simulink model "NonControledLine12"  (R2015b)
settings: configuration reference "ControlConfig" (kept outside this file)
InitFcn:
  | ControlInit;
StopFcn:
  | PlotGridCode;
values from neighbouring files (symbols this model uses):
  c0 = c1/1000    (= 9.22e-13)    [ControlInit.m]
  c1 = 0.922e-9    (= 9.22e-10)    [ControlInit.m]
  Fnom = 50    [ControlInit.m]
  Grid_V = 400e3    (= 400000)    [ControlInit.m]
  L = Vl*Vl/(2*pi*fnom*S)    (= 0.0198943678865)    [XRCalculator.m]
  l0 = l1    (= 0.0013)    [ControlInit.m]
  l1 = 0.0013    [ControlInit.m]
  P_SP = 750e7    (= 7500000000)    [ControlInit.m]
  R = P/(Il*Il)    [XRCalculator.m]
  r0 = r1    (= 0.0731)    [ControlInit.m]
  r1 = 0.0731    [ControlInit.m]
  Ts = 0.02    [ControlInit.m]
  WtF_c0 = WtF_c1/1000    (= 9.22e-09)    [ControlInit.m]
  WtF_c1 = 0.922e-5    (= 9.22e-06)    [ControlInit.m]
  WtF_l0 = WtF_l1    (= 13000)    [ControlInit.m]
  WtF_l1 = 0.0013e7    (= 13000)    [ControlInit.m]
undefined symbols (not defined in the file or in its folder): DiscIntNeverNeededParam
libraries: powerlib x11, simulink x5, powerlib_meascontrol x2
settings Model: Creator=Emilio  LastModifiedBy=Emilio
settings ConfigSetRef: SourceLocation=Base Workspace

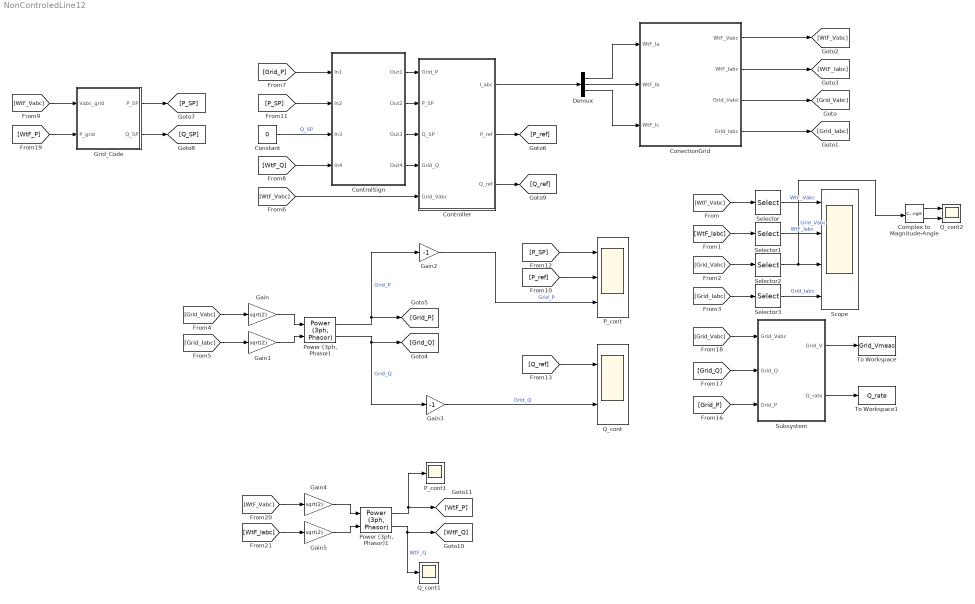
== system NonControledLine12 ==
  Complex to Magnitude-Angle : ComplexToMagnitudeAngle
  ConectionGrid : Subsystem
  Constant : Constant  Value=0
  ControlSign : Subsystem
  Controller : Subsystem
  Demux : Demux  Outputs=3
  Gain{,1,4..5} (4 alike) : Gain  Gain=sqrt(2)
  Gain2 : Gain  Gain=-1
  Gain3 : Gain  Gain=-1
  Grid_Code : Subsystem
  P_cont : Scope  NumInputPorts=3
  P_cont1 : Scope
  "Power (3ph, Phasor)" : powerlib_meascontrol/Measurements/Power (3ph, Phasor)
  "Power (3ph, Phasor)1" : powerlib_meascontrol/Measurements/Power (3ph, Phasor)
  Q_cont : Scope  NumInputPorts=2
  Q_cont1 : Scope
  Q_cont2 : Scope  NumInputPorts=2
  Scope : Scope  NumInputPorts=4
  Selector{,1..3} (4 alike) : Selector  InputPortWidth=3  IndexOptions=Index vector (dialog)  Indices=[1]  OutputSizes=1
  Subsystem : Subsystem
  To Workspace : ToWorkspace  VariableName=Grid_Vmeas  SampleTime=Ts
  To Workspace1 : ToWorkspace  VariableName=Q_rate  SampleTime=-1
  wires:
  ConectionGrid/1(WtF_Vabc) -> [WtF_Vabc]
  ConectionGrid/2(WtF_Iabc) -> [WtF_Iabc]
  ConectionGrid/3(Grid_Vabc) -> [Grid_Vabc]
  ConectionGrid/4(Grid_Iabc) -> [Grid_Iabc]
  [WtF_Vabc] -> Selector/1
  [WtF_Iabc] -> Selector1/1
  [Grid_Vabc] -> Selector2/1
  [Grid_Iabc] -> Selector3/1
  Selector/1 -> Scope/1  "WtF_Vabc"
  Selector1/1 -> Scope/2  "WtF_Iabc"
  Selector2/1 -> Complex to Magnitude-Angle/1, Scope/3  "Grid_Vabc"
  Selector3/1 -> Scope/4  "Grid_Iabc"
  [Grid_Vabc] -> Gain/1
  [Grid_Iabc] -> Gain1/1
  Gain/1 -> "Power (3ph, Phasor)"/1
  Gain1/1 -> "Power (3ph, Phasor)"/2
  "Power (3ph, Phasor)"/1 -> [Grid_P], Gain2/1  "Grid_P"
  "Power (3ph, Phasor)"/2 -> Gain3/1, [Grid_Q]  "Grid_Q"
  [WtF_Vabc] -> Controller/5(Grid_Vabc)
  Controller/1(I_abc) -> Demux/1
  Demux/1 -> ConectionGrid/1(WtF_Ia)
  Demux/2 -> ConectionGrid/2(WtF_Ib)
  Demux/3 -> ConectionGrid/3(WtF_Ic)
  [WtF_Vabc] -> Grid_Code/1(Vabc_grid)
  Gain2/1 -> P_cont/3  "Grid_P"
  Gain3/1 -> Q_cont/2  "Grid_Q"
  Controller/2(P_ref) -> [P_ref]
  [P_ref] -> P_cont/2
  Grid_Code/1(P_SP) -> [P_SP]
  [P_SP] -> P_cont/1
  Grid_Code/2(Q_SP) -> [Q_SP]
  [Q_ref] -> Q_cont/1
  Controller/3(Q_ref) -> [Q_ref]
  [Grid_P] -> Subsystem/3(Grid_P)
  [Grid_Q] -> Subsystem/2(Grid_Q)
  [Grid_Vabc] -> Subsystem/1(Grid_Vabc)
  Subsystem/2(Q_rate) -> To Workspace1/1
  Subsystem/1(Grid_V) -> To Workspace/1
  [WtF_P] -> Grid_Code/2(P_grid)
  [WtF_Vabc] -> Gain4/1
  [WtF_Iabc] -> Gain5/1
  Gain4/1 -> "Power (3ph, Phasor)1"/1
  Gain5/1 -> "Power (3ph, Phasor)1"/2
  "Power (3ph, Phasor)1"/1 -> [WtF_P], P_cont1/1
  "Power (3ph, Phasor)1"/2 -> [WtF_Q], Q_cont1/1  "WtF_Q"
  [P_SP] -> ControlSign/2(In2)
  [WtF_Q] -> ControlSign/4(In4)
  [Grid_P] -> ControlSign/1(In1)
  Constant/1 -> ControlSign/3(In3)  "Q_SP"
  ControlSign/3(Out3) -> Controller/3(Q_SP)
  ControlSign/4(Out4) -> Controller/4(Grid_Q)
  ControlSign/2(Out2) -> Controller/2(P_SP)
  ControlSign/1(Out1) -> Controller/1(Grid_P)
  Complex to Magnitude-Angle/2 -> Q_cont2/2
  Complex to Magnitude-Angle/1 -> Q_cont2/1

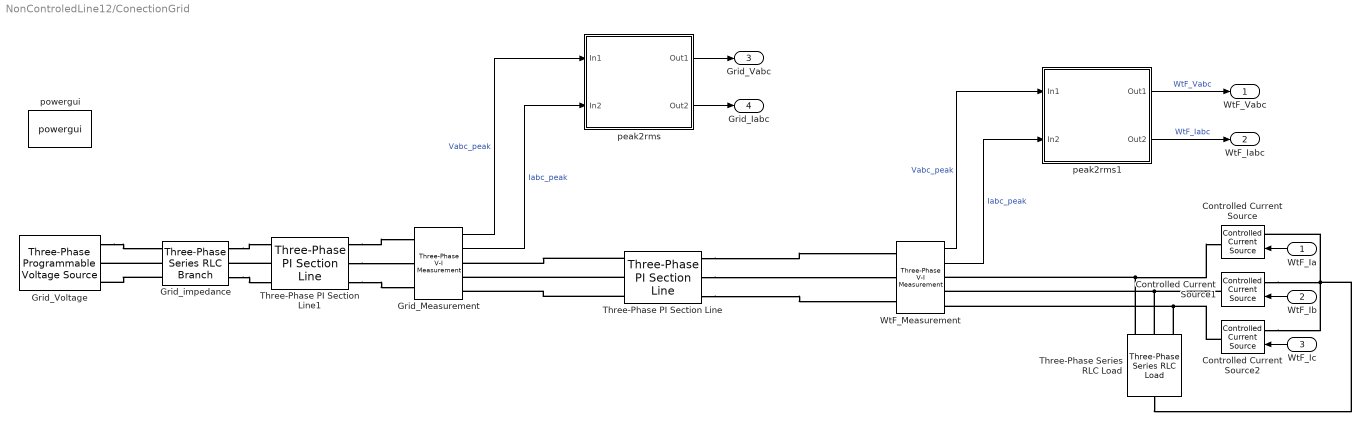
== system NonControledLine12/ConectionGrid ==
  WtF_Ia : Inport
  WtF_Ib : Inport  Port=2
  WtF_Ic : Inport  Port=3
  Controlled Current Source : powerlib/Electrical Sources/Controlled Current Source  Initialize=on  Source_Type=AC  Amplitude=0  Phase=0  Frequency=50  Measurements=None
  Controlled Current Source1 : powerlib/Electrical Sources/Controlled Current Source  Initialize=on  Source_Type=AC  Amplitude=0  Phase=0  Frequency=50  Measurements=None
  Controlled Current Source2 : powerlib/Electrical Sources/Controlled Current Source  Initialize=on  Source_Type=AC  Amplitude=0  Phase=0  Frequency=50  Measurements=None
  Grid_Measurement : powerlib/Measurements/Three-Phase V-I Measurement  VoltageMeasurement=phase-to-ground  SetLabelV=off  LabelV=Vabc  Vpu=off  VpuLL=off  CurrentMeasurement=yes  SetLabelI=off  LabelI=Iabc  Ipu=off  Pbase=100e6  Vbase=500e3  OutputType=Complex  PhasorSimulation=on  PSBequivalent=0
  Grid_Voltage : powerlib/Electrical Sources/Three-Phase Programmable Voltage Source  PositiveSequence="[Grid_V  0 Fnom]"  VariationEntity=None  VariationType=Modulation  VariationTypeAlt=Step  VariationStep=0.025  VariationRate=0.0025  VariationMagnitude=0.05  VariationFrequency=0.05  VariationTiming=[25 35]  VariationPhaseA=off  Amplitudes=[1 0.8 1.2 1.0]  TimeValues=[0 0.1 0.15 0.2]  HarmonicGeneration=off  HarmonicA=[3 0.2 -25 0]  HarmonicB=[2 0.15 35 2]  Timing="[0.05  3]"  BusType=swing  Pref=0  Qref=0  Qmin=-inf  Qmax=inf
  Grid_impedance : powerlib/Elements/Three-Phase Series RLC Branch  LConnTagsString=A|B|C  RConnTagsString=A|B|C  BranchType=RL  Resistance=R  Inductance=L  Capacitance=0  Measurements=None
  Three-Phase PI Section Line : powerlib/Elements/Three-Phase PI Section Line  LConnTagsString=a|b|c  RConnTagsString=A|B|C  Frequency=50  Resistances=[ r1 r0]  Inductances=[ WtF_l1 WtF_l0]  Capacitances=[WtF_c1 WtF_c0]  Length=0.603
  Three-Phase PI Section Line1 : powerlib/Elements/Three-Phase PI Section Line  LConnTagsString=a|b|c  RConnTagsString=A|B|C  Frequency=50  Resistances=[ r1 r0]  Inductances=[l1 l0]  Capacitances=[c1 c0]  Length=0.1219
  Three-Phase Series RLC Load : powerlib/Elements/Three-Phase Series RLC Load  LConnTagsString=A|B|C  RConnTagsString=N  Configuration=Y (neutral)  NominalVoltage=1000  Vabc=[1e3 1e3 1e3]  Vabcp=[1e3 1e3 1e3]  NominalFrequency=50  UnbalancedPower=off  ActivePower=1e-9  InductivePower=0  CapacitivePower=0  Pabc=[10e3 9e3 11e3]  QLabc=[100 90 110]  QCabc=[100 90 110]  Pabcp=[10e3 9e3 11e3]  QLabcp=[100 90 110]  QCabcp=[100 90 110]  Measurements=None  LoadType=constant Z
  WtF_Measurement : powerlib/Measurements/Three-Phase V-I Measurement  VoltageMeasurement=phase-to-ground  SetLabelV=off  LabelV=Vabc  Vpu=off  VpuLL=off  CurrentMeasurement=yes  SetLabelI=off  LabelI=Iabc  Ipu=off  Pbase=100e6  Vbase=500e3  OutputType=Complex  PhasorSimulation=on  PSBequivalent=0
  peak2rms : Subsystem
  peak2rms1 : Subsystem
  powergui : powerlib/powergui  Priority=1  SimulationMode=Phasor  SolverType=Tustin/Backward Euler (TBE)  SampleTime=50e-6  frequency=50  SPID=off  DisableSnubberDevices=off  DisableRonSwitches=off  DisableVfSwitches=off  SwTol=0  DisplayEquations=off  Interpol=off  ExternalGateDelay=off  methode=off  Ts=10  FunctionMessages=off  echomessages=off  HookPort=off  EnableUseOfTLC=off  x0status=blocks  frequencyindice=50  Pbase=100e6  ErrMax=1e-4  Iterations=50  UnitsV=kV  UnitsW=MW  buscounter=0  RestoreLinks=warning  ResistiveCurrentMeasurement=off  Frange=[0:2:500]  Ylog=off  Xlog=on  ShowGrid=off  save=off  variable=ZData  structure=0  ZoomFFT=off  StartTime=0.0  cycles=1  DisplayStyle=1  fundamental=60  FreqAxis=off  MaxFrequency=1000  frequencyindicesteady=1  RmsSteady=1  display=off
  WtF_Vabc : Outport
  WtF_Iabc : Outport  Port=2
  Grid_Vabc : Outport  Port=3
  Grid_Iabc : Outport  Port=4
  wires:
  peak2rms/1(Out1) -> Grid_Vabc/1
  peak2rms/2(Out2) -> Grid_Iabc/1
  Grid_Measurement/2 -> peak2rms/2(In2)  "Iabc_peak"
  Grid_Measurement/1 -> peak2rms/1(In1)  "Vabc_peak"
  WtF_Measurement/2 -> peak2rms1/2(In2)  "Iabc_peak"
  peak2rms1/1(Out1) -> WtF_Vabc/1  "WtF_Vabc"
  peak2rms1/2(Out2) -> WtF_Iabc/1  "WtF_Iabc"
  WtF_Measurement/1 -> peak2rms1/1(In1)  "Vabc_peak"
  WtF_Ic/1 -> Controlled Current Source2/1
  WtF_Ib/1 -> Controlled Current Source1/1
  WtF_Ia/1 -> Controlled Current Source/1
  connections:
  Controlled Current Source/RConn1 -- Three-Phase Series RLC Load/LConn1 -- WtF_Measurement/RConn1
  Controlled Current Source/LConn1 -- Controlled Current Source1/LConn1 -- Three-Phase Series RLC Load/RConn1 -- Controlled Current Source2/LConn1
  Controlled Current Source2/RConn1 -- Three-Phase Series RLC Load/LConn3 -- WtF_Measurement/RConn3
  Controlled Current Source1/RConn1 -- Three-Phase Series RLC Load/LConn2 -- WtF_Measurement/RConn2
  Grid_impedance/LConn2 -- Grid_Voltage/RConn2
  Grid_Voltage/RConn1 -- Grid_impedance/LConn1
  Grid_impedance/LConn3 -- Grid_Voltage/RConn3
  Three-Phase PI Section Line1/RConn2 -- Grid_Measurement/LConn2
  Three-Phase PI Section Line1/LConn2 -- Grid_impedance/RConn2
  Grid_impedance/RConn1 -- Three-Phase PI Section Line1/LConn1
  Grid_impedance/RConn3 -- Three-Phase PI Section Line1/LConn3
  Three-Phase PI Section Line1/RConn1 -- Grid_Measurement/LConn1
  Three-Phase PI Section Line1/RConn3 -- Grid_Measurement/LConn3
  Three-Phase PI Section Line/LConn2 -- Grid_Measurement/RConn2
  Three-Phase PI Section Line/RConn2 -- WtF_Measurement/LConn2
  Three-Phase PI Section Line/RConn1 -- WtF_Measurement/LConn1
  Three-Phase PI Section Line/RConn3 -- WtF_Measurement/LConn3
  Three-Phase PI Section Line/LConn1 -- Grid_Measurement/RConn1
  Three-Phase PI Section Line/LConn3 -- Grid_Measurement/RConn3

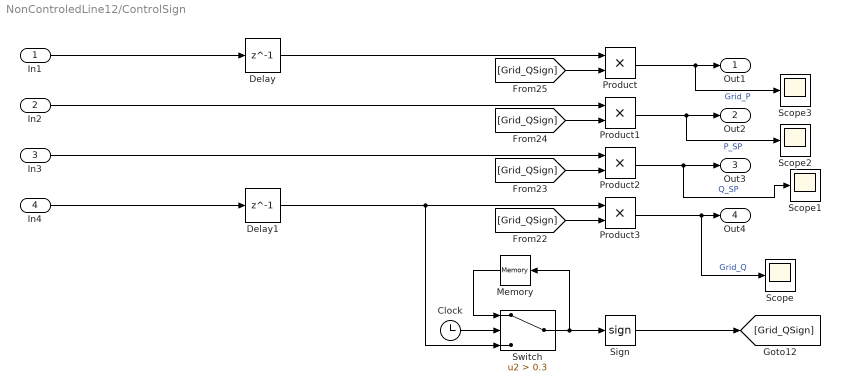
== system NonControledLine12/ControlSign ==
  In1 : Inport
  In2 : Inport  Port=2
  In3 : Inport  Port=3
  In4 : Inport  Port=4
  Clock : Clock
  Delay : Delay  DelayLength=1
  Delay1 : Delay  DelayLength=1
  Memory : Memory
  Product{,1..3} (4 alike) : Product
  Scope{,1..3} (4 alike) : Scope
  Sign : Signum
  Switch : Switch  Criteria=u2 > Threshold  Threshold=0.3
  Out1 : Outport
  Out2 : Outport  Port=2
  Out3 : Outport  Port=3
  Out4 : Outport  Port=4
  wires:
  Sign/1 -> [Grid_QSign]
  In4/1 -> Delay1/1
  In3/1 -> Product2/1
  Clock/1 -> Switch/2
  Memory/1 -> Switch/1
  [Grid_QSign] -> Product1/2
  Product1/1 -> Scope2/1, Out2/1  "P_SP"
  Switch/1 -> Sign/1, Memory/1
  [Grid_QSign] -> Product/2
  In1/1 -> Delay/1
  Product2/1 -> Scope1/1, Out3/1  "Q_SP"
  Product3/1 -> Scope/1, Out4/1  "Grid_Q"
  [Grid_QSign] -> Product2/2
  Product/1 -> Scope3/1, Out1/1  "Grid_P"
  [Grid_QSign] -> Product3/2
  Delay/1 -> Product/1
  In2/1 -> Product1/1
  Delay1/1 -> Product3/1, Switch/3

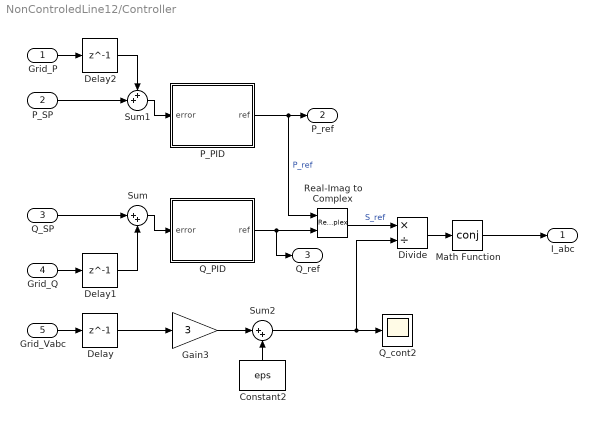
== system NonControledLine12/Controller ==
  Grid_P : Inport
  P_SP : Inport  Port=2
  Q_SP : Inport  Port=3
  Grid_Q : Inport  Port=4
  Grid_Vabc : Inport  Port=5
  Constant2 : Constant  Value=eps
  Delay : Delay  DelayLength=1  InitialCondition=0
  Delay1 : Delay  DelayLength=1  InitialCondition=0
  Delay2 : Delay  DelayLength=1  InitialCondition=0
  Divide : Product  Inputs=*/
  Gain3 : Gain  Gain=3
  Math Function : Math  Operator=conj  SaturateOnIntegerOverflow=on
  P_PID : Subsystem
  Q_PID : Subsystem
  Q_cont2 : Scope
  Real-Imag to Complex : RealImagToComplex
  Sum : Sum  Inputs=|++
  Sum1 : Sum  Inputs=++|
  Sum2 : Sum  Inputs=|++
  I_abc : Outport
  P_ref : Outport  Port=2
  Q_ref : Outport  Port=3
  wires:
  Real-Imag to Complex/1 -> Divide/1  "S_ref"
  Grid_Q/1 -> Delay1/1
  Delay/1 -> Gain3/1
  Grid_Vabc/1 -> Delay/1
  Delay1/1 -> Sum/2
  P_PID/1(ref) -> P_ref/1, Real-Imag to Complex/1  "P_ref"
  Sum1/1 -> P_PID/1(error)
  P_SP/1 -> Sum1/2
  Grid_P/1 -> Delay2/1
  Delay2/1 -> Sum1/1
  Gain3/1 -> Sum2/1
  Constant2/1 -> Sum2/2
  Sum2/1 -> Q_cont2/1, Divide/2
  Divide/1 -> Math Function/1
  Q_PID/1(ref) -> Real-Imag to Complex/2, Q_ref/1
  Q_SP/1 -> Sum/1
  Math Function/1 -> I_abc/1
  Sum/1 -> Q_PID/1(error)

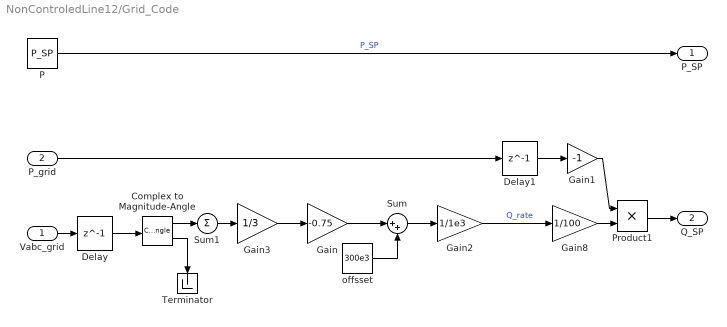
== system NonControledLine12/Grid_Code ==
  Vabc_grid : Inport
  P_grid : Inport  Port=2
  Complex to Magnitude-Angle : ComplexToMagnitudeAngle
  Delay : Delay  DelayLength=1
  Delay1 : Delay  DelayLength=1
  Gain : Gain  Gain=-0.75
  Gain1 : Gain  Gain=-1
  Gain2 : Gain  Gain=1/1e3
  Gain3 : Gain  Gain=1/3
  Gain8 : Gain  Gain=1/100
  P : Constant  Value=P_SP
  Product1 : Product
  Sum : Sum  Inputs=|++
  Sum1 : Sum  Inputs=+
  Terminator : Terminator
  offsset : Constant  Value=300e3
  P_SP : Outport
  Q_SP : Outport  Port=2
  wires:
  P/1 -> P_SP/1  "P_SP"
  Gain/1 -> Sum/1
  offsset/1 -> Sum/2
  Vabc_grid/1 -> Delay/1
  Complex to Magnitude-Angle/1 -> Sum1/1
  Complex to Magnitude-Angle/2 -> Terminator/1
  Delay/1 -> Complex to Magnitude-Angle/1
  Gain2/1 -> Gain8/1  "Q_rate"
  Sum1/1 -> Gain3/1
  Gain3/1 -> Gain/1
  Sum/1 -> Gain2/1
  Gain8/1 -> Product1/2
  Product1/1 -> Q_SP/1
  Gain1/1 -> Product1/1
  Delay1/1 -> Gain1/1
  P_grid/1 -> Delay1/1

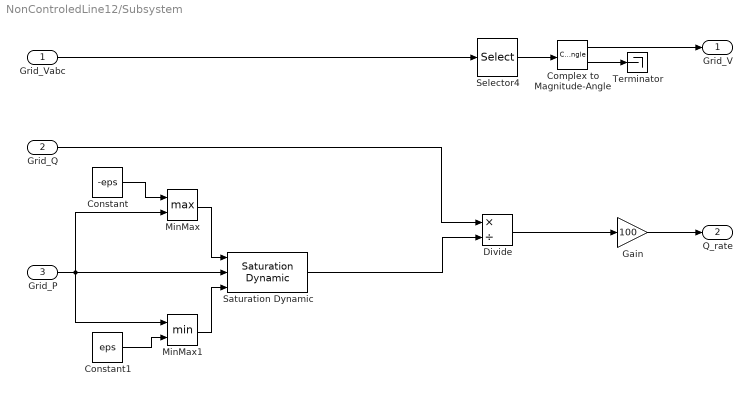
== system NonControledLine12/Subsystem ==
  Grid_Vabc : Inport
  Grid_Q : Inport  Port=2
  Grid_P : Inport  Port=3
  Complex to Magnitude-Angle : ComplexToMagnitudeAngle
  Constant : Constant  Value=-eps
  Constant1 : Constant  Value=eps
  Divide : Product  Inputs=*/
  Gain : Gain  Gain=100
  MinMax : MinMax  Function=max  Inputs=2
  MinMax1 : MinMax  Inputs=2
  Saturation Dynamic : simulink/Discontinuities/Saturation Dynamic  OutMin=[]  OutMax=[]  OutDataTypeStr=Inherit: Same as second input  OutDataType=fixdt(1, 16)  OutScaling=2^-10  DoSatur=off
  Selector4 : Selector  InputPortWidth=3  IndexOptions=Index vector (dialog)  Indices=[1]  OutputSizes=1
  Terminator : Terminator
  Grid_V : Outport
  Q_rate : Outport  Port=2
  wires:
  Divide/1 -> Gain/1
  Selector4/1 -> Complex to Magnitude-Angle/1
  Grid_Vabc/1 -> Selector4/1
  Complex to Magnitude-Angle/2 -> Terminator/1
  Complex to Magnitude-Angle/1 -> Grid_V/1
  Grid_Q/1 -> Divide/1
  Constant/1 -> MinMax/1
  Grid_P/1 -> MinMax/2, MinMax1/1, Saturation Dynamic/2
  MinMax/1 -> Saturation Dynamic/1
  Constant1/1 -> MinMax1/2
  MinMax1/1 -> Saturation Dynamic/3
  Gain/1 -> Q_rate/1
  Saturation Dynamic/1 -> Divide/2

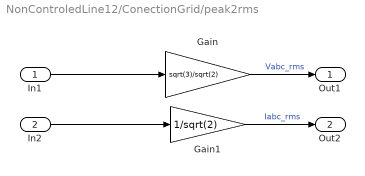
== system NonControledLine12/ConectionGrid/peak2rms ==
  In1 : Inport
  In2 : Inport  Port=2
  Gain : Gain  Gain=sqrt(3)/sqrt(2)
  Gain1 : Gain  Gain=1/sqrt(2)
  Out1 : Outport
  Out2 : Outport  Port=2
  wires:
  Gain/1 -> Out1/1  "Vabc_rms"
  In1/1 -> Gain/1
  Gain1/1 -> Out2/1  "Iabc_rms"
  In2/1 -> Gain1/1

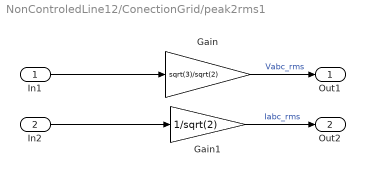
== system NonControledLine12/ConectionGrid/peak2rms1 ==
  In1 : Inport
  In2 : Inport  Port=2
  Gain : Gain  Gain=sqrt(3)/sqrt(2)
  Gain1 : Gain  Gain=1/sqrt(2)
  Out1 : Outport
  Out2 : Outport  Port=2
  wires:
  In2/1 -> Gain1/1
  Gain1/1 -> Out2/1  "Iabc_rms"
  In1/1 -> Gain/1
  Gain/1 -> Out1/1  "Vabc_rms"

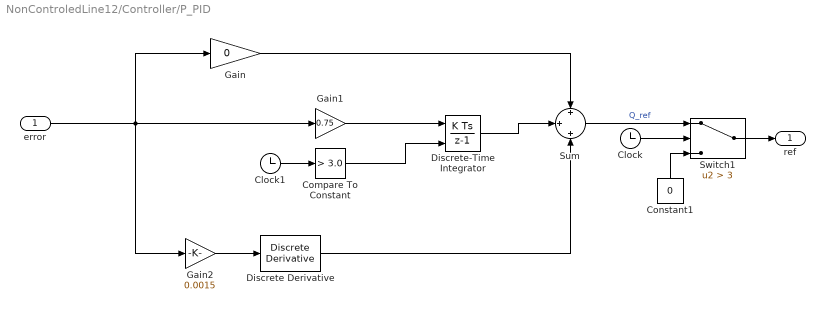
== system NonControledLine12/Controller/P_PID ==
  error : Inport
  Clock : Clock
  Clock1 : Clock
  Compare To Constant : simulink/Logic and Bit Operations/Compare To Constant  relop=>  const=3.0  OutDataTypeStr=boolean
  Constant1 : Constant  Value=0
  Discrete Derivative : simulink/Discrete/Discrete Derivative  gainval=1.0  ICPrevScaledInput=0.0  InputProcessing=Inherited  OutMin=[]  OutMax=[]  OutDataType=fixdt(1, 16)  OutScaling=2^-10  DoSatur=off
  Discrete-Time Integrator : DiscreteIntegrator  ExternalReset=rising  InitialConditionSetting=State (most efficient)  SampleTime=Ts  ICPrevOutput=DiscIntNeverNeededParam  ICPrevScaledInput=DiscIntNeverNeededParam
  Gain : Gain  Gain=0
  Gain1 : Gain  Gain=0.75
  Gain2 : Gain  Gain=0.0015
  Sum : Sum  Inputs=+|+|+
  Switch1 : Switch  Criteria=u2 > Threshold  Threshold=3
  ref : Outport
  wires:
  error/1 -> Gain/1, Gain1/1, Gain2/1
  Discrete Derivative/1 -> Sum/3
  Gain2/1 -> Discrete Derivative/1
  Gain1/1 -> Discrete-Time Integrator/1
  Gain/1 -> Sum/1
  Switch1/1 -> ref/1
  Constant1/1 -> Switch1/3
  Sum/1 -> Switch1/1  "Q_ref"
  Clock/1 -> Switch1/2
  Discrete-Time Integrator/1 -> Sum/2
  Clock1/1 -> Compare To Constant/1
  Compare To Constant/1 -> Discrete-Time Integrator/2

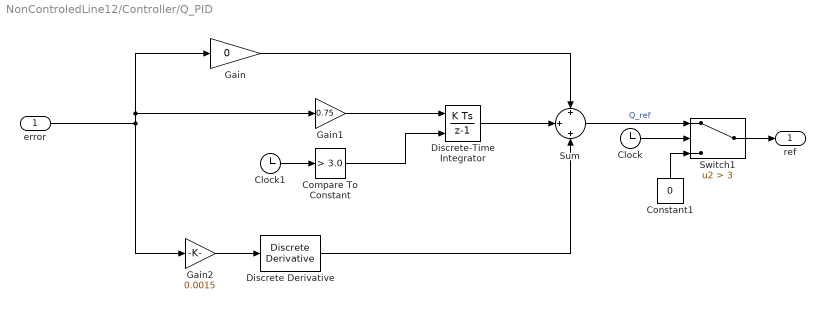
== system NonControledLine12/Controller/Q_PID ==
  error : Inport
  Clock : Clock
  Clock1 : Clock
  Compare To Constant : simulink/Logic and Bit Operations/Compare To Constant  relop=>  const=3.0  OutDataTypeStr=boolean
  Constant1 : Constant  Value=0
  Discrete Derivative : simulink/Discrete/Discrete Derivative  gainval=1.0  ICPrevScaledInput=0.0  InputProcessing=Inherited  OutMin=[]  OutMax=[]  OutDataType=fixdt(1, 16)  OutScaling=2^-10  DoSatur=off
  Discrete-Time Integrator : DiscreteIntegrator  ExternalReset=rising  InitialConditionSetting=State (most efficient)  SampleTime=Ts  ICPrevOutput=DiscIntNeverNeededParam  ICPrevScaledInput=DiscIntNeverNeededParam
  Gain : Gain  Gain=0
  Gain1 : Gain  Gain=0.75
  Gain2 : Gain  Gain=0.0015
  Sum : Sum  Inputs=+|+|+
  Switch1 : Switch  Criteria=u2 > Threshold  Threshold=3
  ref : Outport
  wires:
  Compare To Constant/1 -> Discrete-Time Integrator/2
  Clock1/1 -> Compare To Constant/1
  Discrete-Time Integrator/1 -> Sum/2
  Clock/1 -> Switch1/2
  Sum/1 -> Switch1/1  "Q_ref"
  Constant1/1 -> Switch1/3
  Switch1/1 -> ref/1
  Gain/1 -> Sum/1
  Gain1/1 -> Discrete-Time Integrator/1
  Gain2/1 -> Discrete Derivative/1
  Discrete Derivative/1 -> Sum/3
  error/1 -> Gain1/1, Gain/1, Gain2/1
